simulink model "TRMS_sim_SFV2MPC"  (R2021a)
settings: Solver=VariableStepAuto  StartTime=0.0  StopTime=100  MaxStep=1e-2  RelTol=1e-3
values from neighbouring files (symbols this model uses):
  Ts = 0.01    [BuildGridCustom.m]    (also in workspacesetup.m = 0.02)
  x0 = [0.01,0.010,0.01,0.01,0.01,Thtv0+0.01]    [workspacesetup.m]
undefined symbols (not defined in the file or in its folder): TRMS, uMPC
settings Model: Creator=ariel  LastModifiedBy=ariel

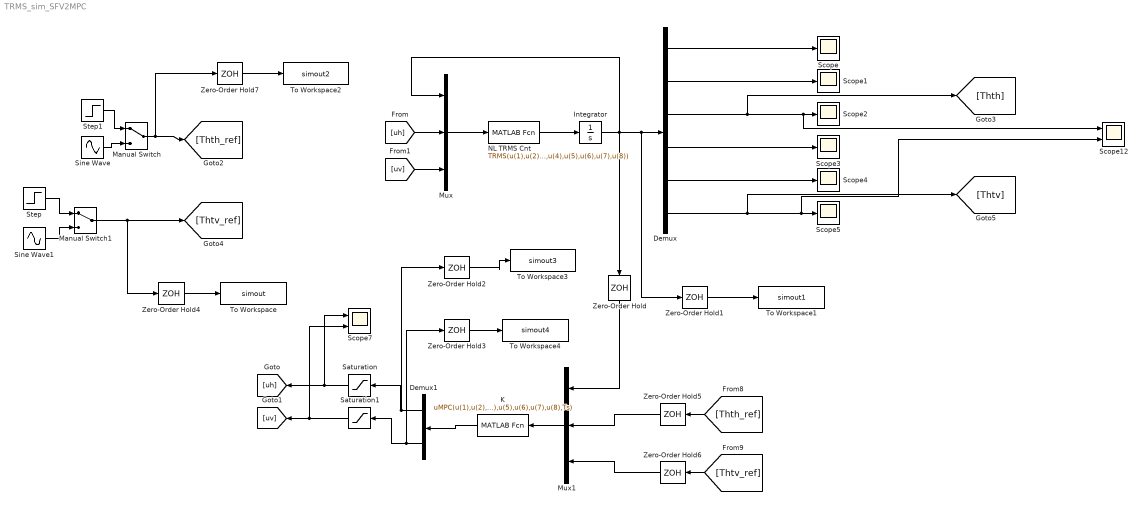
== system TRMS_sim_SFV2MPC ==
  Demux : Demux  Outputs=6
  Demux1 : Demux  Outputs=2
  Integrator : Integrator  InitialCondition=x0
  K : MATLABFcn  MATLABFcn=uMPC(u(1),u(2),u(3),u(4),u(5),u(6),u(7),u(8),Ts)  OutputDimensions=2
  Manual Switch : ManualSwitch
  Manual Switch1 : ManualSwitch
  Mux : Mux  Inputs=3
  Mux1 : Mux  Inputs=3
  NL TRMS Cnt : MATLABFcn  MATLABFcn=TRMS(u(1),u(2),u(3),u(4),u(5),u(6),u(7),u(8))  OutputDimensions=6
  Saturation : Saturate  UpperLimit=2.5  LowerLimit=-2.5
  Saturation1 : Saturate  UpperLimit=2  LowerLimit=-2
  Scope{,1..5} (6 alike) : Scope
  Scope12 : Scope  NumInputPorts=2
  Scope7 : Scope  NumInputPorts=2
  Sine Wave : Sin  Amplitude=0.7  Frequency=2*pi*(1/115)  Phase=0.16  SampleTime=0
  Sine Wave1 : Sin  Amplitude=0.5  Bias=-0.2  Frequency=2*pi*(1/90)  Phase=-0.3  SampleTime=0
  Step : Step  Time=50  Before=-0.4  After=-0.6  SampleTime=1
  Step1 : Step  Time=40  Before=-0.5  After=0.1  SampleTime=1
  To Workspace : ToWorkspace  VariableName=simout  SaveFormat=Timeseries  SampleTime=-1
  To Workspace1 : ToWorkspace  VariableName=simout1  SaveFormat=Timeseries  SampleTime=-1
  To Workspace2 : ToWorkspace  VariableName=simout2  SaveFormat=Timeseries  SampleTime=-1
  To Workspace3 : ToWorkspace  VariableName=simout3  SaveFormat=Timeseries  SampleTime=-1
  To Workspace4 : ToWorkspace  VariableName=simout4  SaveFormat=Timeseries  SampleTime=-1
  Zero-Order Hold{,1..7} (8 alike) : ZeroOrderHold  SampleTime=Ts
  wires:
  NL TRMS Cnt/1 -> Integrator/1
  Mux/1 -> NL TRMS Cnt/1
  Integrator/1 -> Zero-Order Hold/1, Zero-Order Hold1/1, Demux/1, Mux/1
  Demux/1 -> Scope/1
  Demux/5 -> Scope4/1
  Demux/4 -> Scope3/1
  Demux/3 -> [Thth], Scope12/1, Scope2/1
  Demux/2 -> Scope1/1
  K/1 -> Demux1/1
  Demux1/1 -> Zero-Order Hold2/1, Saturation/1
  Demux1/2 -> Zero-Order Hold3/1, Saturation1/1
  [uh] -> Mux/2
  [uv] -> Mux/3
  Demux/6 -> Scope12/2, Scope5/1, [Thtv]
  Saturation/1 -> Scope7/1, [uh]
  Saturation1/1 -> Scope7/2, [uv]
  [Thth_ref] -> Zero-Order Hold5/1
  [Thtv_ref] -> Zero-Order Hold6/1
  Manual Switch/1 -> Zero-Order Hold7/1, [Thth_ref]
  Sine Wave/1 -> Manual Switch/2
  Step1/1 -> Manual Switch/1
  Sine Wave1/1 -> Manual Switch1/2
  Step/1 -> Manual Switch1/1
  Manual Switch1/1 -> Zero-Order Hold4/1, [Thtv_ref]
  Mux1/1 -> K/1
  Zero-Order Hold/1 -> Mux1/1
  Zero-Order Hold5/1 -> Mux1/2
  Zero-Order Hold6/1 -> Mux1/3
  Zero-Order Hold1/1 -> To Workspace1/1
  Zero-Order Hold2/1 -> To Workspace3/1
  Zero-Order Hold3/1 -> To Workspace4/1
  Zero-Order Hold4/1 -> To Workspace/1
  Zero-Order Hold7/1 -> To Workspace2/1
